simulink model "PubIfDecisionTOS_MDL"  (R2020b)
settings: configuration reference "DspaceConfig" (kept outside this file)
PostLoadFcn:
  | if any(exist('dsrtsu_mdlpostloadfcn', 'file') ~= 0), dsrtsu_mdlpostloadfcn('Execute', bdroot); end
InitFcn:
  | , if any(exist('dsmpb_private', 'file') ~= 0), dsmpb_private('dsmpb_mdlclblib', 'Init', bdroot); end,
undefined symbols (not defined in the file or in its folder): C_TOS_ACCEgoRAxletoFbumplength_m, C_TOS_ACCTargetFront_Flag, C_TOS_AEBJAPedObjDxThre_Val, C_TOS_AEBJAPedObjDyThre_Val, C_TOS_AEBJATargetSize_Val, C_TOS_AEBJAVehObjDxThre_Val, C_TOS_AEBJAVehObjDyThre_Val, C_TOS_AEBJuncPedTargetSize_Val, C_TOS_AEBLatObjDxThre_Val, C_TOS_AEBLatPedDyThre_Val, C_TOS_AEBLatTargetSize_Val, C_TOS_AEBLongTargetInEgoFront_Flag, C_TOS_axAbsGround_Parameter, C_TOS_CameraConfirmedFlag, C_TOS_CNsubjWidth, C_TOS_CurrentLaneCoreMinWidth_Val, C_TOS_CutInProb_Val_Zero, C_TOS_CutOutProb_Val_Zero, C_TOS_D2R_Val, C_TOS_DefaultValueObjectToCenterLine_dy, C_TOS_EgoCarWidth_Val, C_TOS_EgoDxRefPoint_m, C_TOS_EgoRAxletoFbumplength_m, C_TOS_HalfWidthVehicle_Con, C_TOS_HWA_CurrentLaneFlag, C_TOS_HWA_LeftLaneFlag, C_TOS_HWA_MovingDir_Vaild, C_TOS_HWA_MovState_Vaild, C_TOS_HWA_RightLaneFlag, C_TOS_LaneLineCourseErrorFront, C_TOS_LaneLineCourseErrorRear, C_TOS_MotorbikeDefaultWidth_m, C_TOS_NumberOfEffectiveTargets, C_TOS_Obj_Age_Val, C_TOS_Objdx_Constraint_Val, C_TOS_ObjectDefaultWidth_m, C_TOS_ObjInCurrentLane_Val, C_TOS_ObjInCurrentLaneValid, C_TOS_ObjInLeftLaneValid, C_TOS_ObjInRightLaneValid, C_TOS_ObjNotInCurrentLane_Val, C_TOS_ObjNotREElementType, C_TOS_ObjPredictDis_dy_ConstantVal_Zeros, C_TOS_ObjToCenterLine_ConstantVal_Zeros, C_TOS_OFMObjIDInvilad_Val, C_TOS_PIL_LatDisCons_Val_zero, C_TOS_PIL_ObjectCutInFlag_b, C_TOS_PIL_ObjectCutOutFlag_b, C_TOS_PIL_ObjLaneProb_al_Val, C_TOS_PP_ObjFusType_FC_Confirm_b, C_TOS_PP_ObjFusType_FC_FR_Confirm_b, C_TOS_PP_ObjFusType_FR_Confirm_b, C_TOS_RE_80BoolDefault_Val, C_TOS_RE_80Single181Default_Val, C_TOS_RE_80Single255Default_Val, C_TOS_RE_80Uint8Default_Val, C_TOS_RE_D2R, C_TOS_RE_D_180_Val, C_TOS_RE_InvalidObjectID_Val, C_TOS_RE_InvalidTargetChainDir_Val ... (+142)
libraries: simulink x1650, TOS_LIB x361, canfdmsglib x14
(part 37 of 69)

== system PubIfDecisionTOS_MDL/TOS_20201112/TOS_2012080320/TOS/ACC/TOS_ACCRightLane/ACC_LeftLane_Target/TOS_ACC_P5/ACC_P5_Targe/ACC_P5_Targe ==
  Object_Fus_Type : Inport
  object_MovingState : Inport  Port=2
  PP_ObjMovingDirSignalProcessing : Inport  Port=3
  Object_HeadingAngle : Inport  Port=4
  Object_DX : Inport  Port=5
  Object_Type : Inport  Port=6
  Object_ObstacleProb : Inport  Port=7
  Object_DY : Inport  Port=8
  PP_ObjFusType_FC_FR_Confirm : Inport  Port=9
  PP_ObjFusType_FR_Confirm : Inport  Port=10
  PP_ObjFusType_FC_Confirm : Inport  Port=11
  Object_VX : Inport  Port=12
  Object_VY : Inport  Port=13
  VIE_EgoVelocity : Inport  Port=14
  SteerWheelAng : Inport  Port=15
  ACC_Target_ID_K1 : Inport  Port=16
  ACC_Target_ID_K2 : Inport  Port=17
  ACC_Target_MovState_K1 : Inport  Port=18
  ACC_Target_MovState_K2 : Inport  Port=19
  ObjectID : Inport  Port=20
  Bus Creator1 : BusCreator  Inputs=20
  Bus Selector : BusSelector  OutputSignals=object_MovingState,PP_ObjFusType_FC_FR_Confirm,PP_ObjFusType_FR_Confirm,PP_ObjFusType_FC_Confirm,ACC_Target_ID_K1,ACC_Target_ID_K2,ACC_Target_MovState_K1,ACC_Target_MovState_K2,ObjectID
  Bus Selector1 : BusSelector  OutputSignals=object_MovingState,PP_ObjMovingDirSignalProcessing,Object_HeadingAngle,Object_VX,Object_VY,VIE_EgoVelocity,SteerWheelAng,ACC_Target_ID_K1,ACC_Target_ID_K2,ACC_Target_MovState_K1,ACC_Target_MovState_K2,ObjectID,Object_Type
  Bus Selector2 : BusSelector  OutputSignals=Object_DX,object_MovingState
  Bus Selector3 : BusSelector  OutputSignals=object_MovingState,Object_Type,ACC_Target_ID_K1,ACC_Target_ID_K2,ACC_Target_MovState_K1,ACC_Target_MovState_K2,ObjectID
  Bus Selector4 : BusSelector  OutputSignals=ACC_Target_ID_K1,ObjectID,Object_ObstacleProb
  Logical Operator4 : Logic  Inputs=5  AllPortsSameDT=off  OutDataTypeStr=boolean
  TOS_ACC_FusionTypeConfirm : Subsystem
  TOS_ACC_ObjTypeConfirm : Subsystem
  TOS_ACC_ObstacleProbConfirm : Subsystem
  TOS_ACC_TargetDxConfirm : Subsystem
  TOS_ACC_TargetMovingDirConfirm : Subsystem
  ACC_P5_TargeConfirm : Outport
  TOS_ACC_FusionType_ObserVale : Outport  Port=2
  TOS_ACC_TrgMovDir_ObserVale : Outport  Port=3
  TOS_ACC_TargetDxConfirm_ObserVale : Outport  Port=4
  TOS_ACC_ObjType_ObserVale : Outport  Port=5
  TOS_ACC_ObstacleProb_ObserVale : Outport  Port=6
  TOS_ACC_TrgMovDirFlag_1_ObserVale : Outport  Port=7
  TOS_ACC_TrgMovDirFlag_2_ObserVale : Outport  Port=8
  TOS_ACC_TrgMovDirFlag_3_ObserVale : Outport  Port=9
  TOS_ACC_TrgMovDirFlag_4_ObserVale : Outport  Port=10
  TOS_ACC_TrgMovDirFlag_5_ObserVale : Outport  Port=11
  TOS_ACC_TrgMovDirFlag_6_ObserVale : Outport  Port=12
  wires:
  TOS_ACC_TargetDxConfirm/1(TOS_ACCTargetInEgoFront) -> [TOS_ACC_TargetDxConfirm_ObserVale], Logical Operator4/3
  TOS_ACC_TargetMovingDirConfirm/1(TOS_ACC_TrgMovDir) -> [TOS_ACC_TrgMovDir_ObserVale], Logical Operator4/2
  Bus Selector2/1 -> TOS_ACC_TargetDxConfirm/1(Object_Dx)  "<Object_DX>"
  TOS_ACC_FusionTypeConfirm/1(TOS_ACCFusionType) -> [TOS_ACC_FusionType_ObserVale], Logical Operator4/1
  TOS_ACC_ObjTypeConfirm/1(TOS_ACCObjType) -> Logical Operator4/4, [TOS_ACC_ObjType_ObserVale]
  Logical Operator4/1 -> ACC_P5_TargeConfirm/1
  [TOS_ACC_FusionType_ObserVale] -> TOS_ACC_FusionType_ObserVale/1
  [TOS_ACC_TrgMovDir_ObserVale] -> TOS_ACC_TrgMovDir_ObserVale/1
  [TOS_ACC_TargetDxConfirm_ObserVale] -> TOS_ACC_TargetDxConfirm_ObserVale/1
  [TOS_ACC_ObjType_ObserVale] -> TOS_ACC_ObjType_ObserVale/1
  [TOS_ACC_ObstacleProb_ObserVale] -> TOS_ACC_ObstacleProb_ObserVale/1
  Bus Selector/1 -> TOS_ACC_FusionTypeConfirm/1(object_MovingState)  "<object_MovingState>"
  Bus Selector1/1 -> TOS_ACC_TargetMovingDirConfirm/1(object_MovingState)  "<object_MovingState>"
  Bus Selector4/3 -> TOS_ACC_ObstacleProbConfirm/3(Object_ObstacleProb)  "<Object_ObstacleProb>"
  TOS_ACC_ObstacleProbConfirm/1(TOS_ACC_ObstacleProb) -> Logical Operator4/5, [TOS_ACC_ObstacleProb_ObserVale]
  Bus Selector/2 -> TOS_ACC_FusionTypeConfirm/2(PP_ObjFusType_FC_FR_Confirm)  "<PP_ObjFusType_FC_FR_Confirm>"
  Bus Selector/3 -> TOS_ACC_FusionTypeConfirm/3(PP_ObjFusType_FR_Confirm)  "<PP_ObjFusType_FR_Confirm>"
  Bus Selector/4 -> TOS_ACC_FusionTypeConfirm/4(PP_ObjFusType_FC_Confirm)  "<PP_ObjFusType_FC_Confirm>"
  Bus Selector/5 -> TOS_ACC_FusionTypeConfirm/5(ACC_Target_ID_K1)  "<ACC_Target_ID_K1>"
  Bus Selector/6 -> TOS_ACC_FusionTypeConfirm/6(ACC_Target_ID_K2)  "<ACC_Target_ID_K2>"
  Bus Selector/9 -> TOS_ACC_FusionTypeConfirm/9(ObjectID)  "<ObjectID>"
  Object_DY/1 -> Bus Creator1/8  "Object_DY"
  PP_ObjFusType_FC_Confirm/1 -> Bus Creator1/11  "PP_ObjFusType_FC_Confirm"
  PP_ObjFusType_FR_Confirm/1 -> Bus Creator1/10  "PP_ObjFusType_FR_Confirm"
  SteerWheelAng/1 -> Bus Creator1/15  "SteerWheelAng"
  ACC_Target_MovState_K1/1 -> Bus Creator1/18  "ACC_Target_MovState_K1"
  ACC_Target_ID_K2/1 -> Bus Creator1/17  "ACC_Target_ID_K2"
  Object_DX/1 -> Bus Creator1/5  "Object_DX"
  Object_ObstacleProb/1 -> Bus Creator1/7  "Object_ObstacleProb"
  ObjectID/1 -> Bus Creator1/20  "ObjectID"
  PP_ObjMovingDirSignalProcessing/1 -> Bus Creator1/3  "PP_ObjMovingDirSignalProcessing"
  VIE_EgoVelocity/1 -> Bus Creator1/14  "VIE_EgoVelocity"
  ACC_Target_ID_K1/1 -> Bus Creator1/16  "ACC_Target_ID_K1"
  Object_HeadingAngle/1 -> Bus Creator1/4  "Object_HeadingAngle"
  PP_ObjFusType_FC_FR_Confirm/1 -> Bus Creator1/9  "PP_ObjFusType_FC_FR_Confirm"
  object_MovingState/1 -> Bus Creator1/2  "object_MovingState"
  ACC_Target_MovState_K2/1 -> Bus Creator1/19  "ACC_Target_MovState_K2"
  Object_VY/1 -> Bus Creator1/13  "Object_VY"
  Object_Fus_Type/1 -> Bus Creator1/1  "Object_Fus_Type1"
  Object_Type/1 -> Bus Creator1/6  "Object_Type"
  Object_VX/1 -> Bus Creator1/12  "Object_VX"
  Bus Creator1/1 -> Bus Selector4/1, Bus Selector3/1, Bus Selector2/1, Bus Selector1/1, Bus Selector/1
  Bus Selector/7 -> TOS_ACC_FusionTypeConfirm/7(ACC_Target_MovState_K1)  "<ACC_Target_MovState_K1>"
  Bus Selector/8 -> TOS_ACC_FusionTypeConfirm/8(ACC_Target_MovState_K2)  "<ACC_Target_MovState_K2>"
  Bus Selector1/2 -> TOS_ACC_TargetMovingDirConfirm/2(PP_ObjMovingDirSignalProcessing)  "<PP_ObjMovingDirSignalProcessing>"
  Bus Selector1/3 -> TOS_ACC_TargetMovingDirConfirm/3(Object_HeadingAngle)  "<Object_HeadingAngle>"
  Bus Selector1/4 -> TOS_ACC_TargetMovingDirConfirm/4(Object_VX)  "<Object_VX>"
  Bus Selector1/5 -> TOS_ACC_TargetMovingDirConfirm/5(Object_VY)  "<Object_VY>"
  Bus Selector1/6 -> TOS_ACC_TargetMovingDirConfirm/6(VIE_EgoVelocity)  "<VIE_EgoVelocity>"
  Bus Selector1/7 -> TOS_ACC_TargetMovingDirConfirm/7(SteerWheelAng)  "<SteerWheelAng>"
  Bus Selector3/1 -> TOS_ACC_ObjTypeConfirm/1(object_MovingState)  "<object_MovingState>"
  Bus Selector3/2 -> TOS_ACC_ObjTypeConfirm/2(Object_Type)  "<Object_Type>"
  Bus Selector4/1 -> TOS_ACC_ObstacleProbConfirm/1(ACC_Target_ID_K1)  "<ACC_Target_ID_K1>"
  Bus Selector4/2 -> TOS_ACC_ObstacleProbConfirm/2(ObjectID)  "<ObjectID>"
  Bus Selector3/3 -> TOS_ACC_ObjTypeConfirm/3(ACC_Target_ID_K1)  "<ACC_Target_ID_K1>"
  Bus Selector3/4 -> TOS_ACC_ObjTypeConfirm/4(ACC_Target_ID_K2)  "<ACC_Target_ID_K2>"
  Bus Selector3/5 -> TOS_ACC_ObjTypeConfirm/5(ACC_Target_MovState_K1)  "<ACC_Target_MovState_K1>"
  Bus Selector3/6 -> TOS_ACC_ObjTypeConfirm/6(ACC_Target_MovState_K2)  "<ACC_Target_MovState_K2>"
  Bus Selector3/7 -> TOS_ACC_ObjTypeConfirm/7(ObjectID)  "<ObjectID>"
  Bus Selector1/8 -> TOS_ACC_TargetMovingDirConfirm/8(ACC_Target_ID_K1)  "<ACC_Target_ID_K1>"
  Bus Selector1/9 -> TOS_ACC_TargetMovingDirConfirm/9(ACC_Target_ID_K2)  "<ACC_Target_ID_K2>"
  Bus Selector1/10 -> TOS_ACC_TargetMovingDirConfirm/10(ACC_Target_MovState_K1)  "<ACC_Target_MovState_K1>"
  Bus Selector1/11 -> TOS_ACC_TargetMovingDirConfirm/11(ACC_Target_MovState_K2)  "<ACC_Target_MovState_K2>"
  Bus Selector1/12 -> TOS_ACC_TargetMovingDirConfirm/12(ObjectID)  "<ObjectID>"
  [TOS_ACC_TrgMovDirFlag_1_ObserVale] -> TOS_ACC_TrgMovDirFlag_1_ObserVale/1
  [TOS_ACC_TrgMovDirFlag_3_ObserVale] -> TOS_ACC_TrgMovDirFlag_3_ObserVale/1
  [TOS_ACC_TrgMovDirFlag_2_ObserVale] -> TOS_ACC_TrgMovDirFlag_2_ObserVale/1
  [TOS_ACC_TrgMovDirFlag_5_ObserVale] -> TOS_ACC_TrgMovDirFlag_5_ObserVale/1
  [TOS_ACC_TrgMovDirFlag_4_ObserVale] -> TOS_ACC_TrgMovDirFlag_4_ObserVale/1
  TOS_ACC_TargetMovingDirConfirm/2(TOS_ACC_TrgMovDirFlag_1_ObserVale) -> [TOS_ACC_TrgMovDirFlag_1_ObserVale]
  TOS_ACC_TargetMovingDirConfirm/3(TOS_ACC_TrgMovDirFlag_2_ObserVale) -> [TOS_ACC_TrgMovDirFlag_2_ObserVale]
  TOS_ACC_TargetMovingDirConfirm/4(TOS_ACC_TrgMovDirFlag_3_ObserVale) -> [TOS_ACC_TrgMovDirFlag_3_ObserVale]
  TOS_ACC_TargetMovingDirConfirm/5(TOS_ACC_TrgMovDirFlag_4_ObserVale) -> [TOS_ACC_TrgMovDirFlag_4_ObserVale]
  TOS_ACC_TargetMovingDirConfirm/6(TOS_ACC_TrgMovDirFlag_5_ObserVale) -> [TOS_ACC_TrgMovDirFlag_5_ObserVale]
  Bus Selector2/2 -> TOS_ACC_TargetDxConfirm/2(object_MovingState)  "<object_MovingState>"
  TOS_ACC_TargetMovingDirConfirm/7(TOS_ACC_TrgMovDirFlag_6_ObserVale) -> [TOS_ACC_TrgMovDirFlag_6_ObserVale]
  [TOS_ACC_TrgMovDirFlag_6_ObserVale] -> TOS_ACC_TrgMovDirFlag_6_ObserVale/1
  Bus Selector1/13 -> TOS_ACC_TargetMovingDirConfirm/13(Object_Type)  "<Object_Type>"

== system PubIfDecisionTOS_MDL/TOS_20201112/TOS_2012080320/TOS/ACC/TOS_ACCRightLane/ACC_Object_PreConfirm/ACC_Object_PreConfirm/ACC_Object_PreConfirm/  ==
  Object_Type : Inport
  Compare To Constant : simulink/Logic and Bit Operations/Compare To Constant  relop===  const=OFM_OBJ_TYPE_E.CAR  OutDataTypeStr=boolean
      settings: AttributesFormatString=OFM_OBJ_TYPE_E.CAR = 2
  Compare To Constant1 : simulink/Logic and Bit Operations/Compare To Constant  relop===  const=OFM_OBJ_TYPE_E.TRUCK  OutDataTypeStr=boolean
      settings: AttributesFormatString=OFM_OBJ_TYPE_E.TRUCK = 3
  Compare To Constant4 : simulink/Logic and Bit Operations/Compare To Constant  relop===  const=OFM_OBJ_TYPE_E.MOTORBIKE  OutDataTypeStr=boolean
      settings: AttributesFormatString=OFM_OBJ_TYPE_E.MOTORBIKE = 4
  Compare To Constant5 : simulink/Logic and Bit Operations/Compare To Constant  relop===  const=OFM_OBJ_TYPE_E.BICYCLE  OutDataTypeStr=boolean
      settings: AttributesFormatString=OFM_OBJ_TYPE_E.BICYCLE = 5
  Data Type Conversion : DataTypeConversion  OutDataTypeStr=Enum: OFM_OBJ_TYPE_E
  Logical Operator1 : Logic  Operator=OR  Inputs=4  AllPortsSameDT=off  OutDataTypeStr=boolean
  TOS_ACC_TargetPre_ObjType : Outport
  wires:
  Logical Operator1/1 -> TOS_ACC_TargetPre_ObjType/1
  Compare To Constant5/1 -> Logical Operator1/4
  Compare To Constant4/1 -> Logical Operator1/3
  Compare To Constant1/1 -> Logical Operator1/2
  Compare To Constant/1 -> Logical Operator1/1
  Data Type Conversion/1 -> Compare To Constant/1, Compare To Constant1/1, Compare To Constant4/1, Compare To Constant5/1
  Object_Type/1 -> Data Type Conversion/1

== system PubIfDecisionTOS_MDL/TOS_20201112/TOS_2012080320/TOS/ACC/TOS_ACCRightLane/ACC_Object_PreConfirm/ACC_Object_PreConfirm/ACC_Object_PreConfirm/Subsystem ==
  PP_ObjFusType_FC_FR_Confirm : Inport
  PP_ObjFusType_FR_Confirm : Inport  Port=2
  PP_ObjFusType_FC_Confirm : Inport  Port=3
  Compare To Constant1 : simulink/Logic and Bit Operations/Compare To Constant  relop===  const=C_TOS_PP_ObjFusType_FC_Confirm_b  OutDataTypeStr=boolean
      settings: AttributesFormatString=C_TOS_PP_ObjFusType_FC_Confirm_b = 1
  Compare To Constant5 : simulink/Logic and Bit Operations/Compare To Constant  relop===  const=C_TOS_PP_ObjFusType_FC_FR_Confirm_b  OutDataTypeStr=boolean
      settings: AttributesFormatString=C_TOS_PP_ObjFusType_FC_FR_Confirm_b = 1
  Compare To Constant6 : simulink/Logic and Bit Operations/Compare To Constant  relop===  const=C_TOS_PP_ObjFusType_FR_Confirm_b  OutDataTypeStr=boolean
      settings: AttributesFormatString=C_TOS_PP_ObjFusType_FR_Confirm_b = 1
  Logical Operator : Logic  Operator=OR  Inputs=3  AllPortsSameDT=off  OutDataTypeStr=boolean
  TOS_ACC_TargetPre_TargetFusionTypeFlag : Outport
  wires:
  Compare To Constant5/1 -> Logical Operator/1
  PP_ObjFusType_FR_Confirm/1 -> Compare To Constant6/1
  PP_ObjFusType_FC_Confirm/1 -> Compare To Constant1/1
  PP_ObjFusType_FC_FR_Confirm/1 -> Compare To Constant5/1
  Compare To Constant6/1 -> Logical Operator/2
  Compare To Constant1/1 -> Logical Operator/3
  Logical Operator/1 -> TOS_ACC_TargetPre_TargetFusionTypeFlag/1

== system PubIfDecisionTOS_MDL/TOS_20201112/TOS_2012080320/TOS/ACC/TOS_ACCRightLane/ACC_Object_PreConfirm/ACC_Object_PreConfirm/ACC_Object_PreConfirm/Subsystem1 ==
  note: 静止目标 、必须有摄像头参与
  PP_ObjFusType_FC_Confirm : Inport
  Obj_MovingState : Inport  Port=2
  Compare To Constant2 : simulink/Logic and Bit Operations/Compare To Constant  relop===  const=OFM_OBJ_MOVINGSTATE_E.UNKNOWN  OutDataTypeStr=boolean
      settings: AttributesFormatString=OFM_OBJ_MOVINGSTATE_E.UNKNOWN = 1
  Compare To Constant3 : simulink/Logic and Bit Operations/Compare To Constant  relop===  const=OFM_OBJ_MOVINGSTATE_E.STATIONARY  OutDataTypeStr=boolean
      settings: AttributesFormatString=OFM_OBJ_MOVINGSTATE_E.STATIONARY = 3
  Compare To Constant5 : simulink/Logic and Bit Operations/Compare To Constant  relop===  const=C_TOS_PP_ObjFusType_FC_Confirm_b  OutDataTypeStr=boolean
      settings: AttributesFormatString=C_TOS_PP_ObjFusType_FC_Confirm_b = 1
  Constant : Constant  OutDataTypeStr=boolean
  Data Type Conversion1 : DataTypeConversion  OutDataTypeStr=Enum: OFM_OBJ_MOVINGSTATE_E
  Logical Operator : Logic  AllPortsSameDT=off  OutDataTypeStr=boolean
  Logical Operator4 : Logic  Operator=OR  AllPortsSameDT=off  OutDataTypeStr=boolean
  Switch : Switch  Criteria=u2 > Threshold
  TOS_ACC_TargetPre_ObjectPassedbyTarget_Flag : Outport
  wires:
  Constant/1 -> Switch/3
  Logical Operator/1 -> Switch/1
  Logical Operator4/1 -> Switch/2, Logical Operator/2
  Compare To Constant2/1 -> Logical Operator4/2
  Compare To Constant5/1 -> Logical Operator/1
  PP_ObjFusType_FC_Confirm/1 -> Compare To Constant5/1
  Data Type Conversion1/1 -> Compare To Constant3/1, Compare To Constant2/1
  Obj_MovingState/1 -> Data Type Conversion1/1
  Compare To Constant3/1 -> Logical Operator4/1
  Switch/1 -> TOS_ACC_TargetPre_ObjectPassedbyTarget_Flag/1

== system PubIfDecisionTOS_MDL/TOS_20201112/TOS_2012080320/TOS/ACC/TOS_ACCRightLane/ACC_Object_PreConfirm/ACC_Object_PreConfirm/ACC_Object_PreConfirm/TOS_ACC_DyConfirm ==
  TOS_ACC_Dy : Inport
  Abs : Abs
  Abs1 : Abs
  Bus Selector3 : BusSelector  OutputSignals=Object_DY,Obj_Dx,Object_ObjType
  Compare To Constant : simulink/Logic and Bit Operations/Compare To Constant  relop===  const=OFM_OBJ_TYPE_E.CAR  OutDataTypeStr=boolean
      settings: AttributesFormatString=OFM_OBJ_TYPE_E.CAR = 2
  Compare To Constant1 : simulink/Logic and Bit Operations/Compare To Constant  relop===  const=OFM_OBJ_TYPE_E.TRUCK  OutDataTypeStr=boolean
      settings: AttributesFormatString=OFM_OBJ_TYPE_E.TRUCK = 3
  Compare To Constant4 : simulink/Logic and Bit Operations/Compare To Constant  relop===  const=OFM_OBJ_TYPE_E.MOTORBIKE  OutDataTypeStr=boolean
      settings: AttributesFormatString=OFM_OBJ_TYPE_E.MOTORBIKE = 4
  Compare To Constant5 : simulink/Logic and Bit Operations/Compare To Constant  relop===  const=OFM_OBJ_TYPE_E.BICYCLE  OutDataTypeStr=boolean
      settings: AttributesFormatString=OFM_OBJ_TYPE_E.BICYCLE = 5
  Data Type Conversion2 : DataTypeConversion  OutDataTypeStr=Enum: OFM_OBJ_TYPE_E
  Logical Operator1 : Logic  Operator=OR  Inputs=4  AllPortsSameDT=off  OutDataTypeStr=boolean
  Logical Operator2 : Logic  Operator=OR  AllPortsSameDT=off  OutDataTypeStr=boolean
  Relational Operator : RelationalOperator  Operator=<=  OutDataTypeStr=boolean  RndMeth=Simplest
  data3 : Lookup_n-D  NumberOfTableDimensions=1  BreakpointsForDimension1=[0,20,40,60,80,100,120,140]  Table=[1.4,1.4,1.3,1.3,1.2,1.2,1.2,1.2]  RndMeth=Simplest  InputSameDT=on
  TOS_ACC_TargetPre_DyConfirm : Outport
  wires:
  Compare To Constant5/1 -> Logical Operator1/4
  Compare To Constant4/1 -> Logical Operator1/3
  Compare To Constant1/1 -> Logical Operator1/2
  Compare To Constant/1 -> Logical Operator1/1
  Bus Selector3/3 -> Data Type Conversion2/1  "<Object_ObjType>"
  Bus Selector3/2 -> Abs/1  "<Obj_Dx>"
  Logical Operator1/1 -> Logical Operator2/2
  Data Type Conversion2/1 -> Compare To Constant1/1, Compare To Constant4/1, Compare To Constant5/1, Compare To Constant/1
  Bus Selector3/1 -> Abs1/1  "<Object_DY>"
  Abs1/1 -> Relational Operator/1
  data3/1 -> Relational Operator/2
  Abs/1 -> data3/1
  Relational Operator/1 -> Logical Operator2/1
  TOS_ACC_Dy/1 -> Bus Selector3/1
  Logical Operator2/1 -> TOS_ACC_TargetPre_DyConfirm/1

== system PubIfDecisionTOS_MDL/TOS_20201112/TOS_2012080320/TOS/AEB/TOS_AEBJunct1105/AEBJunc_Object_Condition/AEBJA_TargetCondition/TOS_AEBJunc_TargetsCondition/AEBJunc_PedTargetCondition ==
  note: 过滤静止目标
  Object_ID : Inport
  PP_ObjFusType_FC_FR_Confirm : Inport  Port=2
  PP_ObjFusType_FR_Confirm : Inport  Port=3
  ObjectType : Inport  Port=4
  Object_Dx : Inport  Port=5
  Object_Dy : Inport  Port=6
  PP_ObjMovingDirSignalProcessing : Inport  Port=7
  Object_HeadingAngle : Inport  Port=8
  Object_VX : Inport  Port=9
  Object_VY : Inport  Port=10
  VIE_EgoVelocity : Inport  Port=11
  psiDtOpt : Inport  Port=12
  axvRefMs2 : Inport  Port=13
  AEBJunc_PedTarget_ObjectID_K1 : Inport  Port=14
  AEBJunc_Target_ObjectType_K1 : Inport  Port=15
  AEBJunc_PedTargetADxDyArea : Subsystem
  AEBJunc_PedTargetFusionTypeJudge : Subsystem
  AEBJunc_PedTargetMoveDir : Subsystem
  AEBJunc_PedTargetObjectTypeFlag : Subsystem
  Chart : Stateflow chart  TreatAsAtomicUnit=on
  Compare To Constant : simulink/Logic and Bit Operations/Compare To Constant  relop===  const=true  OutDataTypeStr=boolean
  Logical Operator : Logic  Inputs=4  AllPortsSameDT=off  OutDataTypeStr=boolean
  Terminator : Terminator
  TOS_AEBJunc_PedTargetsDx : Outport
  AEBJunc_PedTargetFusionType_observal : Outport  Port=2
  AEBJunc_PedTargetObjectType_observal : Outport  Port=3
  AEBJunc_PedTargetDXDY_observal : Outport  Port=4
  AEBJunc_PedTargetMovDir_observal : Outport  Port=5
  wires:
  AEBJunc_PedTargetMoveDir/1(TOS_AEBJuncTargetMovDirFlg) -> [AEBJuncPedMovDirFlg], Logical Operator/4
  Object_HeadingAngle/1 -> AEBJunc_PedTargetMoveDir/4(Object_HeadingAngle)
  PP_ObjFusType_FC_FR_Confirm/1 -> AEBJunc_PedTargetFusionTypeJudge/1(PP_ObjFusType_FC_FR_Confirm)
  [Object_Dx] -> AEBJunc_PedTargetMoveDir/2(Object_Dx)  "Object_Dx"
  [Object_Dx] -> Chart/6(Object_Dx)
  Object_Dx/1 -> [Object_Dx], AEBJunc_PedTargetADxDyArea/1(Object_Dx)
  [AEBJunc_PedFusionTypeFlag] -> AEBJunc_PedTargetFusionType_observal/1
  AEBJunc_PedTargetADxDyArea/1(TOS_AEBJunc_DxDyAreaFlag) -> Logical Operator/3, [AEBJunc_PedDxDyAreaFlag]
  Logical Operator/1 -> Compare To Constant/1
  Chart/1(TOS_AEBJunc_TargetsDx) -> TOS_AEBJunc_PedTargetsDx/1
  [AEBJunc_PedObjectTypeFlag] -> AEBJunc_PedTargetObjectType_observal/1
  PP_ObjMovingDirSignalProcessing/1 -> AEBJunc_PedTargetMoveDir/3(PP_ObjMovingDirSignalProcessing)
  psiDtOpt/1 -> Chart/3(psiDtOpt)
  PP_ObjFusType_FR_Confirm/1 -> AEBJunc_PedTargetFusionTypeJudge/2(PP_ObjFusType_FR_Confirm)
  Object_VY/1 -> [Object_Vy], AEBJunc_PedTargetMoveDir/6(Object_VY)
  VIE_EgoVelocity/1 -> AEBJunc_PedTargetMoveDir/7(VIE_EgoVelocity)
  AEBJunc_PedTargetFusionTypeJudge/1(AEBJunc_TargetFusionTypeFlag) -> [AEBJunc_PedFusionTypeFlag], Logical Operator/1
  Object_VX/1 -> AEBJunc_PedTargetMoveDir/5(Object_VX)
  Object_Dy/1 -> AEBJunc_PedTargetMoveDir/1(Object_Dy), AEBJunc_PedTargetADxDyArea/2(Object_Dy)
  AEBJunc_PedTargetObjectTypeFlag/1(AEBJunc_PedTargetObjectTypeFlag) -> [AEBJunc_PedObjectTypeFlag], Logical Operator/2
  [AEBJuncPedMovDirFlg] -> AEBJunc_PedTargetMovDir_observal/1
  axvRefMs2/1 -> AEBJunc_PedTargetMoveDir/8(axvRefMs2)
  ObjectType/1 -> AEBJunc_PedTargetObjectTypeFlag/1(ObjectType)
  [AEBJunc_PedDxDyAreaFlag] -> AEBJunc_PedTargetDXDY_observal/1
  [Object_Vy] -> Chart/5(Object_Vy)
  Compare To Constant/1 -> Chart/1(AEBJunc_TargetCondition)
  AEBJunc_Target_ObjectType_K1/1 -> Terminator/1
  Object_ID/1 -> [Object_ID], AEBJunc_PedTargetObjectTypeFlag/3(ObjectID)
  AEBJunc_PedTarget_ObjectID_K1/1 -> [AEBJunc_PedTarget_ObjectID_K1], AEBJunc_PedTargetObjectTypeFlag/2(AEBLat_Target_ID_K1)
  [Object_ID] -> Chart/2(Object_ID)
  [AEBJunc_PedTarget_ObjectID_K1] -> Chart/4(AEBJunc_Target_ObjectID_K1)

== system PubIfDecisionTOS_MDL/TOS_20201112/TOS_2012080320/TOS/AEB/TOS_AEBJunct1105/AEBJunc_Object_Condition/AEBJA_TargetCondition/TOS_AEBJunc_TargetsCondition/AEBJunc_VehTargetCondition ==
  note: 过滤静止目标
  Object_ID : Inport
  PP_ObjFusType_FC_FR_Confirm : Inport  Port=2
  PP_ObjFusType_FR_Confirm : Inport  Port=3
  ObjectType : Inport  Port=4
  Object_Dx : Inport  Port=5
  Object_Dy : Inport  Port=6
  PP_ObjMovingDirSignalProcessing : Inport  Port=7
  Object_HeadingAngle : Inport  Port=8
  Object_VX : Inport  Port=9
  Object_VY : Inport  Port=10
  VIE_EgoVelocity : Inport  Port=11
  psiDtOpt : Inport  Port=12
  axvRefMs2 : Inport  Port=13
  AEBJunc_VehTarget_ObjectID_K1 : Inport  Port=14
  AEBJunc_Target_ObjectType_K1 : Inport  Port=15
  Object_MovingState : Inport  Port=16
  AEBJunc_VehTargetADxDyArea : Subsystem
  AEBJunc_VehTargetFusionTypeJudge : Subsystem
  AEBJunc_VehTargetObjectTypeFlag : Subsystem
  Chart : Stateflow chart  Commented=on  TreatAsAtomicUnit=on
  Compare To Constant : simulink/Logic and Bit Operations/Compare To Constant  relop===  const=true  OutDataTypeStr=boolean
  Constant : Constant  Value=255  OutDataTypeStr=single
  From5 : From  Commented=on  GotoTag=Object_Vy
  From7 : From  Commented=on  GotoTag=Object_Dx
  From8 : From  Commented=on  GotoTag=AEBJunc_VehTarget_ObjectID_K1
  From9 : From  Commented=on  GotoTag=Object_ID
  Goto5 : Goto  Commented=on  GotoTag=Object_Vy
  Goto7 : Goto  Commented=on  GotoTag=AEBJunc_VehTarget_ObjectID_K1
  Goto8 : Goto  Commented=on  GotoTag=Object_ID
  Logical Operator : Logic  Inputs=5  AllPortsSameDT=off  OutDataTypeStr=boolean
  Subsystem : Subsystem
  Switch : Switch  Criteria=u2 ~= 0
  TOS_AEBJunc_VehTargetMoveDir : Subsystem
  Terminator : Terminator
  TOS_AEBJunc_VehTargetsDx : Outport
  AEBJunc_VehTargetFusionType_observal : Outport  Port=2
  AEBJunc_VehTargetObjectType_observal : Outport  Port=3
  AEBJunc_VehTargetDXDY_observal : Outport  Port=4
  AEBJunc_VehTargetMovDir_observal : Outport  Port=5
  AEBJunc_VehTargetMovState_observal : Outport  Port=6
  wires:
  AEBJunc_Target_ObjectType_K1/1 -> Terminator/1
  From5/1 -> Chart/5(Object_Vy)
  [TOS_AEBJunc_VehDxDyAreaFlag] -> AEBJunc_VehTargetDXDY_observal/1
  ObjectType/1 -> AEBJunc_VehTargetObjectTypeFlag/1(ObjectType)
  axvRefMs2/1 -> TOS_AEBJunc_VehTargetMoveDir/7(axvRefMs2)
  [TOS_AEBJuncVehMovDirFlg] -> AEBJunc_VehTargetMovDir_observal/1
  AEBJunc_VehTargetObjectTypeFlag/1(AEBJunc_VehTargetObjectTypeFlag) -> Logical Operator/2, [AEBJunc_VehObjectTypeFlag]
  Object_Dy/1 -> AEBJunc_VehTargetADxDyArea/2(Object_Dy)
  Object_VX/1 -> TOS_AEBJunc_VehTargetMoveDir/4(Object_VX)
  AEBJunc_VehTargetFusionTypeJudge/1(AEBJunc_VehTargetFusionTypeFlag) -> Logical Operator/1, [AEBJunc_VehFusionTypeFlag]
  VIE_EgoVelocity/1 -> TOS_AEBJunc_VehTargetMoveDir/6(VIE_EgoVelocity)
  Object_VY/1 -> TOS_AEBJunc_VehTargetMoveDir/5(Object_VY), Goto5/1
  PP_ObjFusType_FR_Confirm/1 -> AEBJunc_VehTargetFusionTypeJudge/2(PP_ObjFusType_FR_Confirm)
  psiDtOpt/1 -> Chart/3(psiDtOpt)
  PP_ObjMovingDirSignalProcessing/1 -> TOS_AEBJunc_VehTargetMoveDir/2(PP_ObjMovingDirSignalProcessing)
  [AEBJunc_VehObjectTypeFlag] -> AEBJunc_VehTargetObjectType_observal/1
  Logical Operator/1 -> Compare To Constant/1
  AEBJunc_VehTargetADxDyArea/1(TOS_AEBJunc_VehDxDyAreaFlag) -> [TOS_AEBJunc_VehDxDyAreaFlag], Logical Operator/3
  [AEBJunc_VehFusionTypeFlag] -> AEBJunc_VehTargetFusionType_observal/1
  Object_Dx/1 -> AEBJunc_VehTargetADxDyArea/1(Object_Dx), [Object_Dx]
  From7/1 -> Chart/6(Object_Dx)
  [Object_Dx] -> TOS_AEBJunc_VehTargetMoveDir/1(Object_Dx)  "Object_Dx"
  PP_ObjFusType_FC_FR_Confirm/1 -> AEBJunc_VehTargetFusionTypeJudge/1(PP_ObjFusType_FC_FR_Confirm)
  Object_HeadingAngle/1 -> TOS_AEBJunc_VehTargetMoveDir/3(Object_HeadingAngle)
  TOS_AEBJunc_VehTargetMoveDir/1(TOS_AEBJuncVehTargetMovDirFlg) -> Logical Operator/4, [TOS_AEBJuncVehMovDirFlg]  "TOS_AEBJunc_VehTargetMovDir"
  Object_MovingState/1 -> Subsystem/1(Object_MovingState)
  Subsystem/1(TOS_AEBJuncVehTargetMovStateFlg) -> Logical Operator/5, [TOS_AEBJuncVehMovStateFlg]
  [TOS_AEBJuncVehMovStateFlg] -> AEBJunc_VehTargetMovState_observal/1
  Object_ID/1 -> Goto8/1, AEBJunc_VehTargetObjectTypeFlag/3(ObjectID)
  AEBJunc_VehTarget_ObjectID_K1/1 -> Goto7/1, AEBJunc_VehTargetObjectTypeFlag/2(AEBJunc_VehTarget_ID_K1)
  From8/1 -> Chart/4(AEBJunc_Target_ObjectID_K1)
  From9/1 -> Chart/2(Object_ID)
  [Object_Dx] -> Switch/1
  Compare To Constant/1 -> Switch/2
  Constant/1 -> Switch/3
  Switch/1 -> TOS_AEBJunc_VehTargetsDx/1

== system PubIfDecisionTOS_MDL/TOS_20201112/TOS_2012080320/TOS/AEB/TOS_AEBJunct1105/AEBJunc_Object_Condition1/AEBJA_TargetCondition/TOS_AEBJunc_TargetsCondition/AEBJunc_PedTargetCondition ==
  note: 过滤静止目标
  Object_ID : Inport
  PP_ObjFusType_FC_FR_Confirm : Inport  Port=2
  PP_ObjFusType_FR_Confirm : Inport  Port=3
  ObjectType : Inport  Port=4
  Object_Dx : Inport  Port=5
  Object_Dy : Inport  Port=6
  PP_ObjMovingDirSignalProcessing : Inport  Port=7
  Object_HeadingAngle : Inport  Port=8
  Object_VX : Inport  Port=9
  Object_VY : Inport  Port=10
  VIE_EgoVelocity : Inport  Port=11
  psiDtOpt : Inport  Port=12
  axvRefMs2 : Inport  Port=13
  AEBJunc_PedTarget_ObjectID_K1 : Inport  Port=14
  AEBJunc_Target_ObjectType_K1 : Inport  Port=15
  AEBJunc_PedTargetADxDyArea : Subsystem
  AEBJunc_PedTargetFusionTypeJudge : Subsystem
  AEBJunc_PedTargetMoveDir : Subsystem
  AEBJunc_PedTargetObjectTypeFlag : Subsystem
  Chart : Stateflow chart  TreatAsAtomicUnit=on
  Compare To Constant : simulink/Logic and Bit Operations/Compare To Constant  relop===  const=true  OutDataTypeStr=boolean
  Logical Operator : Logic  Inputs=4  AllPortsSameDT=off  OutDataTypeStr=boolean
  Terminator : Terminator
  TOS_AEBJunc_PedTargetsDx : Outport
  AEBJunc_PedTargetFusionType_observal : Outport  Port=2
  AEBJunc_PedTargetObjectType_observal : Outport  Port=3
  AEBJunc_PedTargetDXDY_observal : Outport  Port=4
  AEBJunc_PedTargetMovDir_observal : Outport  Port=5
  wires:
  [AEBJunc_PedTarget_ObjectID_K1] -> Chart/4(AEBJunc_Target_ObjectID_K1)
  [Object_ID] -> Chart/2(Object_ID)
  AEBJunc_PedTarget_ObjectID_K1/1 -> AEBJunc_PedTargetObjectTypeFlag/2(AEBLat_Target_ID_K1), [AEBJunc_PedTarget_ObjectID_K1]
  Object_ID/1 -> AEBJunc_PedTargetObjectTypeFlag/3(ObjectID), [Object_ID]
  AEBJunc_Target_ObjectType_K1/1 -> Terminator/1
  Compare To Constant/1 -> Chart/1(AEBJunc_TargetCondition)
  [Object_Vy] -> Chart/5(Object_Vy)
  [AEBJunc_PedDxDyAreaFlag] -> AEBJunc_PedTargetDXDY_observal/1
  ObjectType/1 -> AEBJunc_PedTargetObjectTypeFlag/1(ObjectType)
  axvRefMs2/1 -> AEBJunc_PedTargetMoveDir/8(axvRefMs2)
  [AEBJuncPedMovDirFlg] -> AEBJunc_PedTargetMovDir_observal/1
  AEBJunc_PedTargetObjectTypeFlag/1(AEBJunc_PedTargetObjectTypeFlag) -> Logical Operator/2, [AEBJunc_PedObjectTypeFlag]
  Object_Dy/1 -> AEBJunc_PedTargetADxDyArea/2(Object_Dy), AEBJunc_PedTargetMoveDir/1(Object_Dy)
  Object_VX/1 -> AEBJunc_PedTargetMoveDir/5(Object_VX)
  AEBJunc_PedTargetFusionTypeJudge/1(AEBJunc_TargetFusionTypeFlag) -> Logical Operator/1, [AEBJunc_PedFusionTypeFlag]
  VIE_EgoVelocity/1 -> AEBJunc_PedTargetMoveDir/7(VIE_EgoVelocity)
  Object_VY/1 -> AEBJunc_PedTargetMoveDir/6(Object_VY), [Object_Vy]
  PP_ObjFusType_FR_Confirm/1 -> AEBJunc_PedTargetFusionTypeJudge/2(PP_ObjFusType_FR_Confirm)
  psiDtOpt/1 -> Chart/3(psiDtOpt)
  PP_ObjMovingDirSignalProcessing/1 -> AEBJunc_PedTargetMoveDir/3(PP_ObjMovingDirSignalProcessing)
  [AEBJunc_PedObjectTypeFlag] -> AEBJunc_PedTargetObjectType_observal/1
  Chart/1(TOS_AEBJunc_TargetsDx) -> TOS_AEBJunc_PedTargetsDx/1
  Logical Operator/1 -> Compare To Constant/1
  AEBJunc_PedTargetADxDyArea/1(TOS_AEBJunc_DxDyAreaFlag) -> [AEBJunc_PedDxDyAreaFlag], Logical Operator/3
  [AEBJunc_PedFusionTypeFlag] -> AEBJunc_PedTargetFusionType_observal/1
  Object_Dx/1 -> AEBJunc_PedTargetADxDyArea/1(Object_Dx), [Object_Dx]
  [Object_Dx] -> Chart/6(Object_Dx)
  [Object_Dx] -> AEBJunc_PedTargetMoveDir/2(Object_Dx)  "Object_Dx"
  PP_ObjFusType_FC_FR_Confirm/1 -> AEBJunc_PedTargetFusionTypeJudge/1(PP_ObjFusType_FC_FR_Confirm)
  Object_HeadingAngle/1 -> AEBJunc_PedTargetMoveDir/4(Object_HeadingAngle)
  AEBJunc_PedTargetMoveDir/1(TOS_AEBJuncTargetMovDirFlg) -> Logical Operator/4, [AEBJuncPedMovDirFlg]

== system PubIfDecisionTOS_MDL/TOS_20201112/TOS_2012080320/TOS/AEB/TOS_AEBJunct1105/AEBJunc_Object_Condition1/AEBJA_TargetCondition/TOS_AEBJunc_TargetsCondition/AEBJunc_VehTargetCondition ==
  note: 过滤静止目标
  Object_ID : Inport
  PP_ObjFusType_FC_FR_Confirm : Inport  Port=2
  PP_ObjFusType_FR_Confirm : Inport  Port=3
  ObjectType : Inport  Port=4
  Object_Dx : Inport  Port=5
  Object_Dy : Inport  Port=6
  PP_ObjMovingDirSignalProcessing : Inport  Port=7
  Object_HeadingAngle : Inport  Port=8
  Object_VX : Inport  Port=9
  Object_VY : Inport  Port=10
  VIE_EgoVelocity : Inport  Port=11
  psiDtOpt : Inport  Port=12
  axvRefMs2 : Inport  Port=13
  AEBJunc_VehTarget_ObjectID_K1 : Inport  Port=14
  AEBJunc_Target_ObjectType_K1 : Inport  Port=15
  Object_MovingState : Inport  Port=16
  AEBJunc_VehTargetADxDyArea : Subsystem
  AEBJunc_VehTargetFusionTypeJudge : Subsystem
  AEBJunc_VehTargetObjectTypeFlag : Subsystem
  Chart : Stateflow chart  TreatAsAtomicUnit=on
  Compare To Constant : simulink/Logic and Bit Operations/Compare To Constant  relop===  const=true  OutDataTypeStr=boolean
  Logical Operator : Logic  Inputs=5  AllPortsSameDT=off  OutDataTypeStr=boolean
  Subsystem : Subsystem
  TOS_AEBJunc_VehTargetMoveDir : Subsystem
  Terminator : Terminator
  TOS_AEBJunc_VehTargetsDx : Outport
  AEBJunc_VehTargetFusionType_observal : Outport  Port=2
  AEBJunc_VehTargetObjectType_observal : Outport  Port=3
  AEBJunc_VehTargetDXDY_observal : Outport  Port=4
  AEBJunc_VehTargetMovDir_observal : Outport  Port=5
  AEBJunc_VehTargetMovState_observal : Outport  Port=6
  wires:
  [Object_ID] -> Chart/2(Object_ID)
  [AEBJunc_VehTarget_ObjectID_K1] -> Chart/4(AEBJunc_Target_ObjectID_K1)
  AEBJunc_VehTarget_ObjectID_K1/1 -> AEBJunc_VehTargetObjectTypeFlag/2(AEBJunc_VehTarget_ID_K1), [AEBJunc_VehTarget_ObjectID_K1]
  Object_ID/1 -> AEBJunc_VehTargetObjectTypeFlag/3(ObjectID), [Object_ID]
  [TOS_AEBJuncVehMovStateFlg] -> AEBJunc_VehTargetMovState_observal/1
  Subsystem/1(TOS_AEBJuncVehTargetMovStateFlg) -> [TOS_AEBJuncVehMovStateFlg], Logical Operator/5
  Object_MovingState/1 -> Subsystem/1(Object_MovingState)
  TOS_AEBJunc_VehTargetMoveDir/1(TOS_AEBJuncVehTargetMovDirFlg) -> [TOS_AEBJuncVehMovDirFlg], Logical Operator/4  "TOS_AEBJunc_VehTargetMovDir"
  Object_HeadingAngle/1 -> TOS_AEBJunc_VehTargetMoveDir/3(Object_HeadingAngle)
  PP_ObjFusType_FC_FR_Confirm/1 -> AEBJunc_VehTargetFusionTypeJudge/1(PP_ObjFusType_FC_FR_Confirm)
  [Object_Dx] -> TOS_AEBJunc_VehTargetMoveDir/1(Object_Dx)  "Object_Dx"
  [Object_Dx] -> Chart/6(Object_Dx)
  Object_Dx/1 -> [Object_Dx], AEBJunc_VehTargetADxDyArea/1(Object_Dx)
  [AEBJunc_VehFusionTypeFlag] -> AEBJunc_VehTargetFusionType_observal/1
  AEBJunc_VehTargetADxDyArea/1(TOS_AEBJunc_VehDxDyAreaFlag) -> Logical Operator/3, [TOS_AEBJunc_VehDxDyAreaFlag]
  Logical Operator/1 -> Compare To Constant/1
  Chart/1(TOS_AEBJunc_TargetsDx) -> TOS_AEBJunc_VehTargetsDx/1
  [AEBJunc_VehObjectTypeFlag] -> AEBJunc_VehTargetObjectType_observal/1
  PP_ObjMovingDirSignalProcessing/1 -> TOS_AEBJunc_VehTargetMoveDir/2(PP_ObjMovingDirSignalProcessing)
  psiDtOpt/1 -> Chart/3(psiDtOpt)
  PP_ObjFusType_FR_Confirm/1 -> AEBJunc_VehTargetFusionTypeJudge/2(PP_ObjFusType_FR_Confirm)
  Object_VY/1 -> [Object_Vy], TOS_AEBJunc_VehTargetMoveDir/5(Object_VY)
  VIE_EgoVelocity/1 -> TOS_AEBJunc_VehTargetMoveDir/6(VIE_EgoVelocity)
  AEBJunc_VehTargetFusionTypeJudge/1(AEBJunc_VehTargetFusionTypeFlag) -> [AEBJunc_VehFusionTypeFlag], Logical Operator/1
  Object_VX/1 -> TOS_AEBJunc_VehTargetMoveDir/4(Object_VX)
  Object_Dy/1 -> AEBJunc_VehTargetADxDyArea/2(Object_Dy)
  AEBJunc_VehTargetObjectTypeFlag/1(AEBJunc_VehTargetObjectTypeFlag) -> [AEBJunc_VehObjectTypeFlag], Logical Operator/2
  [TOS_AEBJuncVehMovDirFlg] -> AEBJunc_VehTargetMovDir_observal/1
  axvRefMs2/1 -> TOS_AEBJunc_VehTargetMoveDir/7(axvRefMs2)
  ObjectType/1 -> AEBJunc_VehTargetObjectTypeFlag/1(ObjectType)
  [TOS_AEBJunc_VehDxDyAreaFlag] -> AEBJunc_VehTargetDXDY_observal/1
  [Object_Vy] -> Chart/5(Object_Vy)
  Compare To Constant/1 -> Chart/1(AEBJunc_TargetCondition)
  AEBJunc_Target_ObjectType_K1/1 -> Terminator/1

== system PubIfDecisionTOS_MDL/TOS_20201112/TOS_2012080320/TOS/AEB/TOS_AEBJunct_20201208/AEBJunc_Object_Condition/AEBJA_TargetCondition/TOS_AEBJunc_TargetsCondition/AEBJunc_PedTargetCondition ==
  note: 过滤静止目标
  Object_ID : Inport
  PP_ObjFusType_FC_FR_Confirm : Inport  Port=2
  PP_ObjFusType_FR_Confirm : Inport  Port=3
  ObjectType : Inport  Port=4
  Object_Dx : Inport  Port=5
  Object_Dy : Inport  Port=6
  PP_ObjMovingDirSignalProcessing : Inport  Port=7
  Object_HeadingAngle : Inport  Port=8
  Object_VX : Inport  Port=9
  Object_VY : Inport  Port=10
  VIE_EgoVelocity : Inport  Port=11
  psiDtOpt : Inport  Port=12
  axvRefMs2 : Inport  Port=13
  AEBJunc_PedTarget_ObjectID_K1 : Inport  Port=14
  AEBJunc_Target_ObjectType_K1 : Inport  Port=15
  AEBJunc_PedTargetADxDyArea : Subsystem
  AEBJunc_PedTargetFusionTypeJudge : Subsystem
  AEBJunc_PedTargetMoveDir : Subsystem
  AEBJunc_PedTargetObjectTypeFlag : Subsystem
  Chart : Stateflow chart  TreatAsAtomicUnit=on
  Compare To Constant : simulink/Logic and Bit Operations/Compare To Constant  relop===  const=true  OutDataTypeStr=boolean
  Logical Operator : Logic  Inputs=4  AllPortsSameDT=off  OutDataTypeStr=boolean
  Terminator : Terminator
  TOS_AEBJunc_PedTargetsDx : Outport
  AEBJunc_PedTargetFusionType_observal : Outport  Port=2
  AEBJunc_PedTargetObjectType_observal : Outport  Port=3
  AEBJunc_PedTargetDXDY_observal : Outport  Port=4
  AEBJunc_PedTargetMovDir_observal : Outport  Port=5
  wires:
  AEBJunc_PedTargetMoveDir/1(TOS_AEBJuncTargetMovDirFlg) -> [AEBJuncPedMovDirFlg], Logical Operator/4
  Object_HeadingAngle/1 -> AEBJunc_PedTargetMoveDir/4(Object_HeadingAngle)
  PP_ObjFusType_FC_FR_Confirm/1 -> AEBJunc_PedTargetFusionTypeJudge/1(PP_ObjFusType_FC_FR_Confirm)
  [Object_Dx] -> AEBJunc_PedTargetMoveDir/2(Object_Dx)  "Object_Dx"
  [Object_Dx] -> Chart/6(Object_Dx)
  Object_Dx/1 -> [Object_Dx], AEBJunc_PedTargetADxDyArea/1(Object_Dx)
  [AEBJunc_PedFusionTypeFlag] -> AEBJunc_PedTargetFusionType_observal/1
  AEBJunc_PedTargetADxDyArea/1(TOS_AEBJunc_DxDyAreaFlag) -> Logical Operator/3, [AEBJunc_PedDxDyAreaFlag]
  Logical Operator/1 -> Compare To Constant/1
  Chart/1(TOS_AEBJunc_TargetsDx) -> TOS_AEBJunc_PedTargetsDx/1
  [AEBJunc_PedObjectTypeFlag] -> AEBJunc_PedTargetObjectType_observal/1
  PP_ObjMovingDirSignalProcessing/1 -> AEBJunc_PedTargetMoveDir/3(PP_ObjMovingDirSignalProcessing)
  psiDtOpt/1 -> Chart/3(psiDtOpt)
  PP_ObjFusType_FR_Confirm/1 -> AEBJunc_PedTargetFusionTypeJudge/2(PP_ObjFusType_FR_Confirm)
  Object_VY/1 -> [Object_Vy], AEBJunc_PedTargetMoveDir/6(Object_VY)
  VIE_EgoVelocity/1 -> AEBJunc_PedTargetMoveDir/7(VIE_EgoVelocity)
  AEBJunc_PedTargetFusionTypeJudge/1(AEBJunc_TargetFusionTypeFlag) -> [AEBJunc_PedFusionTypeFlag], Logical Operator/1
  Object_VX/1 -> AEBJunc_PedTargetMoveDir/5(Object_VX)
  Object_Dy/1 -> AEBJunc_PedTargetMoveDir/1(Object_Dy), AEBJunc_PedTargetADxDyArea/2(Object_Dy)
  AEBJunc_PedTargetObjectTypeFlag/1(AEBJunc_PedTargetObjectTypeFlag) -> [AEBJunc_PedObjectTypeFlag], Logical Operator/2
  [AEBJuncPedMovDirFlg] -> AEBJunc_PedTargetMovDir_observal/1
  axvRefMs2/1 -> AEBJunc_PedTargetMoveDir/8(axvRefMs2)
  ObjectType/1 -> AEBJunc_PedTargetObjectTypeFlag/1(ObjectType)
  [AEBJunc_PedDxDyAreaFlag] -> AEBJunc_PedTargetDXDY_observal/1
  [Object_Vy] -> Chart/5(Object_Vy)
  Compare To Constant/1 -> Chart/1(AEBJunc_TargetCondition)
  AEBJunc_Target_ObjectType_K1/1 -> Terminator/1
  Object_ID/1 -> [Object_ID], AEBJunc_PedTargetObjectTypeFlag/3(ObjectID)
  AEBJunc_PedTarget_ObjectID_K1/1 -> [AEBJunc_PedTarget_ObjectID_K1], AEBJunc_PedTargetObjectTypeFlag/2(AEBLat_Target_ID_K1)
  [Object_ID] -> Chart/2(Object_ID)
  [AEBJunc_PedTarget_ObjectID_K1] -> Chart/4(AEBJunc_Target_ObjectID_K1)
  [Object_ID] -> AEBJunc_PedTargetMoveDir/10(ObjectID)
  [AEBJunc_PedTarget_ObjectID_K1] -> AEBJunc_PedTargetMoveDir/9(AEBJunc_Target_ID_K1)

== system PubIfDecisionTOS_MDL/TOS_20201112/TOS_2012080320/TOS/AEB/TOS_AEBJunct_20201208/AEBJunc_Object_Condition/AEBJA_TargetCondition/TOS_AEBJunc_TargetsCondition/AEBJunc_VehTargetCondition ==
  note: 过滤静止目标
  Object_ID : Inport
  PP_ObjFusType_FC_FR_Confirm : Inport  Port=2
  PP_ObjFusType_FR_Confirm : Inport  Port=3
  ObjectType : Inport  Port=4
  Object_Dx : Inport  Port=5
  Object_Dy : Inport  Port=6
  PP_ObjMovingDirSignalProcessing : Inport  Port=7
  Object_HeadingAngle : Inport  Port=8
  Object_VX : Inport  Port=9
  Object_VY : Inport  Port=10
  VIE_EgoVelocity : Inport  Port=11
  psiDtOpt : Inport  Port=12
  axvRefMs2 : Inport  Port=13
  AEBJunc_VehTarget_ObjectID_K1 : Inport  Port=14
  AEBJunc_Target_ObjectType_K1 : Inport  Port=15
  Object_MovingState : Inport  Port=16
  AEBJunc_VehTargetADxDyArea : Subsystem
  AEBJunc_VehTargetFusionTypeJudge : Subsystem
  AEBJunc_VehTargetObjectTypeFlag : Subsystem
  Chart : Stateflow chart  Commented=on  TreatAsAtomicUnit=on
  Compare To Constant : simulink/Logic and Bit Operations/Compare To Constant  relop===  const=true  OutDataTypeStr=boolean
  Constant : Constant  Value=255  OutDataTypeStr=single
  From5 : From  Commented=on  GotoTag=Object_Vy
  From7 : From  Commented=on  GotoTag=Object_Dx
  From8 : From  Commented=on  GotoTag=AEBJunc_VehTarget_ObjectID_K1
  From9 : From  Commented=on  GotoTag=Object_ID
  Goto5 : Goto  Commented=on  GotoTag=Object_Vy
  Logical Operator : Logic  Inputs=5  AllPortsSameDT=off  OutDataTypeStr=boolean
  Subsystem : Subsystem
  Switch : Switch  Criteria=u2 ~= 0
  TOS_AEBJunc_VehTargetMoveDir : Subsystem
  Terminator : Terminator
  TOS_AEBJunc_VehTargetsDx : Outport
  AEBJunc_VehTargetFusionType_observal : Outport  Port=2
  AEBJunc_VehTargetObjectType_observal : Outport  Port=3
  AEBJunc_VehTargetDXDY_observal : Outport  Port=4
  AEBJunc_VehTargetMovDir_observal : Outport  Port=5
  AEBJunc_VehTargetMovState_observal : Outport  Port=6
  wires:
  AEBJunc_Target_ObjectType_K1/1 -> Terminator/1
  From5/1 -> Chart/5(Object_Vy)
  [TOS_AEBJunc_VehDxDyAreaFlag] -> AEBJunc_VehTargetDXDY_observal/1
  ObjectType/1 -> AEBJunc_VehTargetObjectTypeFlag/1(ObjectType)
  axvRefMs2/1 -> TOS_AEBJunc_VehTargetMoveDir/7(axvRefMs2)
  [TOS_AEBJuncVehMovDirFlg] -> AEBJunc_VehTargetMovDir_observal/1
  AEBJunc_VehTargetObjectTypeFlag/1(AEBJunc_VehTargetObjectTypeFlag) -> Logical Operator/2, [AEBJunc_VehObjectTypeFlag]
  Object_Dy/1 -> AEBJunc_VehTargetADxDyArea/2(Object_Dy)
  Object_VX/1 -> TOS_AEBJunc_VehTargetMoveDir/4(Object_VX)
  AEBJunc_VehTargetFusionTypeJudge/1(AEBJunc_VehTargetFusionTypeFlag) -> Logical Operator/1, [AEBJunc_VehFusionTypeFlag]
  VIE_EgoVelocity/1 -> TOS_AEBJunc_VehTargetMoveDir/6(VIE_EgoVelocity)
  Object_VY/1 -> Goto5/1, TOS_AEBJunc_VehTargetMoveDir/5(Object_VY)
  PP_ObjFusType_FR_Confirm/1 -> AEBJunc_VehTargetFusionTypeJudge/2(PP_ObjFusType_FR_Confirm)
  psiDtOpt/1 -> Chart/3(psiDtOpt)
  PP_ObjMovingDirSignalProcessing/1 -> TOS_AEBJunc_VehTargetMoveDir/2(PP_ObjMovingDirSignalProcessing)
  [AEBJunc_VehObjectTypeFlag] -> AEBJunc_VehTargetObjectType_observal/1
  Logical Operator/1 -> Compare To Constant/1
  AEBJunc_VehTargetADxDyArea/1(TOS_AEBJunc_VehDxDyAreaFlag) -> [TOS_AEBJunc_VehDxDyAreaFlag], Logical Operator/3
  [AEBJunc_VehFusionTypeFlag] -> AEBJunc_VehTargetFusionType_observal/1
  Object_Dx/1 -> AEBJunc_VehTargetADxDyArea/1(Object_Dx), [Object_Dx]
  From7/1 -> Chart/6(Object_Dx)
  [Object_Dx] -> TOS_AEBJunc_VehTargetMoveDir/1(Object_Dx)  "Object_Dx"
  PP_ObjFusType_FC_FR_Confirm/1 -> AEBJunc_VehTargetFusionTypeJudge/1(PP_ObjFusType_FC_FR_Confirm)
  Object_HeadingAngle/1 -> TOS_AEBJunc_VehTargetMoveDir/3(Object_HeadingAngle)
  TOS_AEBJunc_VehTargetMoveDir/1(TOS_AEBJuncVehTargetMovDirFlg) -> Logical Operator/4, [TOS_AEBJuncVehMovDirFlg]  "TOS_AEBJunc_VehTargetMovDir"
  Object_MovingState/1 -> Subsystem/1(Object_MovingState)
  Subsystem/1(TOS_AEBJuncVehTargetMovStateFlg) -> Logical Operator/5, [TOS_AEBJuncVehMovStateFlg]
  [TOS_AEBJuncVehMovStateFlg] -> AEBJunc_VehTargetMovState_observal/1
  Object_ID/1 -> [Object_ID], AEBJunc_VehTargetObjectTypeFlag/3(ObjectID)
  AEBJunc_VehTarget_ObjectID_K1/1 -> [AEBJunc_VehTarget_ObjectID_K1], AEBJunc_VehTargetObjectTypeFlag/2(AEBJunc_VehTarget_ID_K1)
  From8/1 -> Chart/4(AEBJunc_Target_ObjectID_K1)
  From9/1 -> Chart/2(Object_ID)
  [Object_Dx] -> Switch/1
  Compare To Constant/1 -> Switch/2
  Constant/1 -> Switch/3
  Switch/1 -> TOS_AEBJunc_VehTargetsDx/1
  [AEBJunc_VehTarget_ObjectID_K1] -> TOS_AEBJunc_VehTargetMoveDir/8(AEBJunc_Target_ID_K1)
  [Object_ID] -> TOS_AEBJunc_VehTargetMoveDir/9(ObjectID)

== system PubIfDecisionTOS_MDL/TOS_20201112/TOS_2012080320/TOS/AEB/TOS_AEBJunct_20201208/AEBJunc_Object_Condition1/AEBJA_TargetCondition/TOS_AEBJunc_TargetsCondition/AEBJunc_PedTargetCondition ==
  note: 过滤静止目标
  Object_ID : Inport
  PP_ObjFusType_FC_FR_Confirm : Inport  Port=2
  PP_ObjFusType_FR_Confirm : Inport  Port=3
  ObjectType : Inport  Port=4
  Object_Dx : Inport  Port=5
  Object_Dy : Inport  Port=6
  PP_ObjMovingDirSignalProcessing : Inport  Port=7
  Object_HeadingAngle : Inport  Port=8
  Object_VX : Inport  Port=9
  Object_VY : Inport  Port=10
  VIE_EgoVelocity : Inport  Port=11
  psiDtOpt : Inport  Port=12
  axvRefMs2 : Inport  Port=13
  AEBJunc_PedTarget_ObjectID_K1 : Inport  Port=14
  AEBJunc_Target_ObjectType_K1 : Inport  Port=15
  AEBJunc_PedTargetADxDyArea : Subsystem
  AEBJunc_PedTargetFusionTypeJudge : Subsystem
  AEBJunc_PedTargetMoveDir : Subsystem
  AEBJunc_PedTargetObjectTypeFlag : Subsystem
  Chart : Stateflow chart  TreatAsAtomicUnit=on
  Compare To Constant : simulink/Logic and Bit Operations/Compare To Constant  relop===  const=true  OutDataTypeStr=boolean
  Logical Operator : Logic  Inputs=4  AllPortsSameDT=off  OutDataTypeStr=boolean
  Terminator : Terminator
  TOS_AEBJunc_PedTargetsDx : Outport
  AEBJunc_PedTargetFusionType_observal : Outport  Port=2
  AEBJunc_PedTargetObjectType_observal : Outport  Port=3
  AEBJunc_PedTargetDXDY_observal : Outport  Port=4
  AEBJunc_PedTargetMovDir_observal : Outport  Port=5
  wires:
  [AEBJunc_PedTarget_ObjectID_K1] -> Chart/4(AEBJunc_Target_ObjectID_K1)
  [Object_ID] -> Chart/2(Object_ID)
  AEBJunc_PedTarget_ObjectID_K1/1 -> AEBJunc_PedTargetObjectTypeFlag/2(AEBLat_Target_ID_K1), [AEBJunc_PedTarget_ObjectID_K1]
  Object_ID/1 -> AEBJunc_PedTargetObjectTypeFlag/3(ObjectID), [Object_ID]
  AEBJunc_Target_ObjectType_K1/1 -> Terminator/1
  Compare To Constant/1 -> Chart/1(AEBJunc_TargetCondition)
  [Object_Vy] -> Chart/5(Object_Vy)
  [AEBJunc_PedDxDyAreaFlag] -> AEBJunc_PedTargetDXDY_observal/1
  ObjectType/1 -> AEBJunc_PedTargetObjectTypeFlag/1(ObjectType)
  axvRefMs2/1 -> AEBJunc_PedTargetMoveDir/8(axvRefMs2)
  [AEBJuncPedMovDirFlg] -> AEBJunc_PedTargetMovDir_observal/1
  AEBJunc_PedTargetObjectTypeFlag/1(AEBJunc_PedTargetObjectTypeFlag) -> Logical Operator/2, [AEBJunc_PedObjectTypeFlag]
  Object_Dy/1 -> AEBJunc_PedTargetADxDyArea/2(Object_Dy), AEBJunc_PedTargetMoveDir/1(Object_Dy)
  Object_VX/1 -> AEBJunc_PedTargetMoveDir/5(Object_VX)
  AEBJunc_PedTargetFusionTypeJudge/1(AEBJunc_TargetFusionTypeFlag) -> Logical Operator/1, [AEBJunc_PedFusionTypeFlag]
  VIE_EgoVelocity/1 -> AEBJunc_PedTargetMoveDir/7(VIE_EgoVelocity)
  Object_VY/1 -> AEBJunc_PedTargetMoveDir/6(Object_VY), [Object_Vy]
  PP_ObjFusType_FR_Confirm/1 -> AEBJunc_PedTargetFusionTypeJudge/2(PP_ObjFusType_FR_Confirm)
  psiDtOpt/1 -> Chart/3(psiDtOpt)
  PP_ObjMovingDirSignalProcessing/1 -> AEBJunc_PedTargetMoveDir/3(PP_ObjMovingDirSignalProcessing)
  [AEBJunc_PedObjectTypeFlag] -> AEBJunc_PedTargetObjectType_observal/1
  Chart/1(TOS_AEBJunc_TargetsDx) -> TOS_AEBJunc_PedTargetsDx/1
  Logical Operator/1 -> Compare To Constant/1
  AEBJunc_PedTargetADxDyArea/1(TOS_AEBJunc_DxDyAreaFlag) -> [AEBJunc_PedDxDyAreaFlag], Logical Operator/3
  [AEBJunc_PedFusionTypeFlag] -> AEBJunc_PedTargetFusionType_observal/1
  Object_Dx/1 -> AEBJunc_PedTargetADxDyArea/1(Object_Dx), [Object_Dx]
  [Object_Dx] -> Chart/6(Object_Dx)
  [Object_Dx] -> AEBJunc_PedTargetMoveDir/2(Object_Dx)  "Object_Dx"
  PP_ObjFusType_FC_FR_Confirm/1 -> AEBJunc_PedTargetFusionTypeJudge/1(PP_ObjFusType_FC_FR_Confirm)
  Object_HeadingAngle/1 -> AEBJunc_PedTargetMoveDir/4(Object_HeadingAngle)
  AEBJunc_PedTargetMoveDir/1(TOS_AEBJuncTargetMovDirFlg) -> Logical Operator/4, [AEBJuncPedMovDirFlg]
